simulink model "Lab4"  (R2023b)
settings: Solver=FixedStepDiscrete  StartTime=0.0  StopTime=50  FixedStep=0.01  RelTol=1e-3
settings Model: Creator=cosmi  LastModifiedBy=MrLove

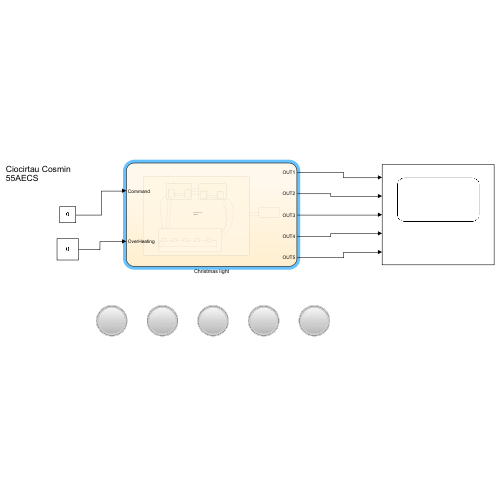
[thumbnail: Simulink's stored preview of the top-level diagram]
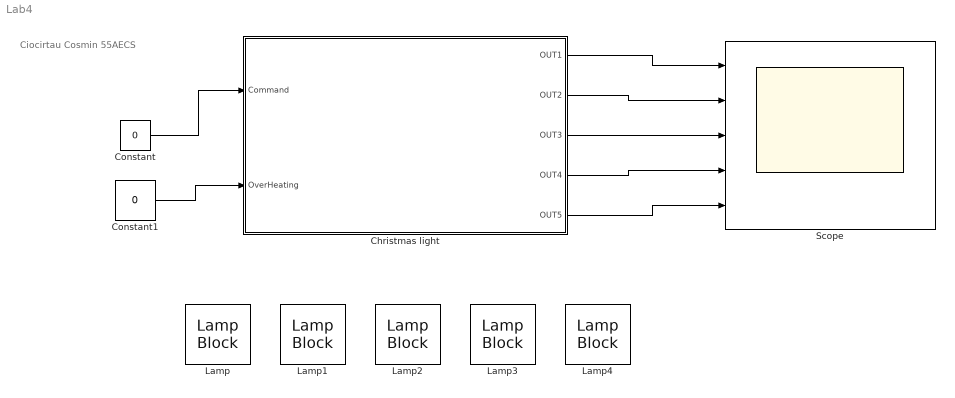
== system Lab4 ==
  note: Ciocirtau Cosmin
      | 55AECS
  Christmas light : Stateflow chart  TreatAsAtomicUnit=on
  Constant : Constant  Value=0
  Constant1 : Constant  Value=0
  Lamp{,1..4} (5 alike) : LampBlock  LabelPosition=Hide
  Scope : Scope  NumInputPorts=5
  wires:
  Christmas light/1(OUT1) -> Scope/1
  Christmas light/2(OUT2) -> Scope/2
  Christmas light/3(OUT3) -> Scope/3
  Christmas light/4(OUT4) -> Scope/4
  Christmas light/5(OUT5) -> Scope/5
  Constant/1 -> Christmas light/1(Command)
  Constant1/1 -> Christmas light/2(OverHeating)

== stateflow chart Lab4/Christmas light ==
  state Working
    state Mode1
      state Mode1_ON
        en:
        OUT1 = 100;
        OUT2 = 100;
        OUT3 = 100;
        OUT4 = 100;
        OUT5 = 100;
      state Mode1_OFF
        en:
        OUT1 = 0;
        OUT2 = 0;
        OUT3 = 0;
        OUT4 = 0;
        OUT5 = 0;
      (default) -> Mode1_ON
      Mode1_ON -> Mode1_OFF : [after(200,msec)]
      Mode1_OFF -> Mode1_ON : [after(200,msec)]
    state Mode2
      en:
      OUT1 = 0;
      OUT2 = 0;
      OUT3 = 0;
      OUT4 = 0;
      OUT5 = 0;
      state Mode2_INC
      state Mode2_DEC
        du:
        OUT1 = OUT1 - 1/3;
        OUT2 = OUT2 - 1/3;
        OUT3 = OUT3 - 1/3;
        OUT4 = OUT4 - 1/3;
        OUT5 = OUT5 - 1/3;
      (default) -> Mode2_INC
      Mode2_INC -> Mode2_INC [order 2] : [after(30,msec)]
          | {OUT1 = OUT1 + 1;
          | OUT2 =  OUT2 + 1;
          | OUT3 =  OUT3 + 1;
          | OUT4 =  OUT4 + 1;
          | OUT5 =  OUT5 + 1;}
      Mode2_INC -> Mode2_DEC [order 1] : [OUT1>=100]
      Mode2_DEC -> Mode2_INC : [OUT1<=0]
    note: 1/3 x 0.01s (model settings)
    note: Ciocirtau Cosmin
        | 55AECS
    state Mode_3
      state Mode3_1
        en:
        OUT1 = 100;
        OUT2 =  0;
        OUT3 =  0;
        OUT4 =  0;
        OUT5 =  0;
      state Mode3_2
        en:
        OUT1 = 0;
        OUT2 =  100;
        OUT3 =  0;
        OUT4 =  0;
        OUT5 =  0;
      state Mode3_3
        en:
        OUT1 = 0;
        OUT2 =  0;
        OUT3 =  100;
        OUT4 =  0;
        OUT5 =  0;
      state Mode3_4
        en:
        OUT1 = 0;
        OUT2 =  0;
        OUT3 =  0;
        OUT4 =  100;
        OUT5 =  0;
      state Mode3_5
        en:
        OUT1 = 0;
        OUT2 =  0;
        OUT3 =  0;
        OUT4 =  0;
        OUT5 =  100;
      (default) -> Mode3_1
      (junction 45) -> Mode3_1
      Mode3_5 -> (junction 42) : [after(250, msec)]
      Mode3_1 -> Mode3_2 : [after(250, msec)]
      Mode3_2 -> Mode3_3 : [after(250, msec)]
      Mode3_3 -> Mode3_4 : [after(250, msec)]
      Mode3_4 -> Mode3_5 : [after(250, msec)]
      (junction 44) -> (junction 45)
      (junction 42) -> (junction 43)
      (junction 43) -> (junction 44)
    (default) -> Mode1
    Mode1 -> Mode2 [order 1] : [Command  == 0 && after(10, sec)]
    Mode2 -> Mode1 [order 3] : [Command == 1]
    Mode1 -> Mode2 [order 2] : [Command == 2]
    Mode_3 -> Mode1 [order 1] : [Command  == 1]
    Mode2 -> Mode_3 [order 1] : [Command  == 0 && after(10, sec)]
    Mode1 -> Mode_3 [order 3] : [Command == 3]
    Mode_3 -> Mode1 [order 2] : [Command  == 0 && after(10, sec)]
    Mode_3 -> Mode2 [order 3] : [Command  == 2]
    Mode2 -> Mode_3 [order 2] : [Comand  == 3]
  state Disabled
    en:
    OUT1 = 0;
    OUT2 = 0;
    OUT3 = 0;
    OUT4 = 0;
    OUT5 = 0;
  (default) -> Working
  Working -> Disabled : [OverHeating == true]
  Disabled -> Working : [after(15,sec) && OverHeating == false]
  data: OUT1 output; OUT2 output; OUT3 output; OUT4 output; OUT5 output; Command input; OverHeating input
